simulink library "OSEM_WD"  (Simulink 7.5)
settings: Solver=ode45  StartTime=0.0  StopTime=10.0  RelTol=1e-3
libraries: cdsFunctionCall x3, cdsEpicsOut x2, cdsTrueRMS x1
settings Model: Creator=controls  LastModifiedBy=controls

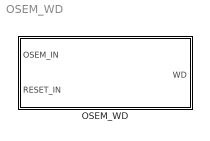
== system OSEM_WD ==
  OSEM_WD : Subsystem

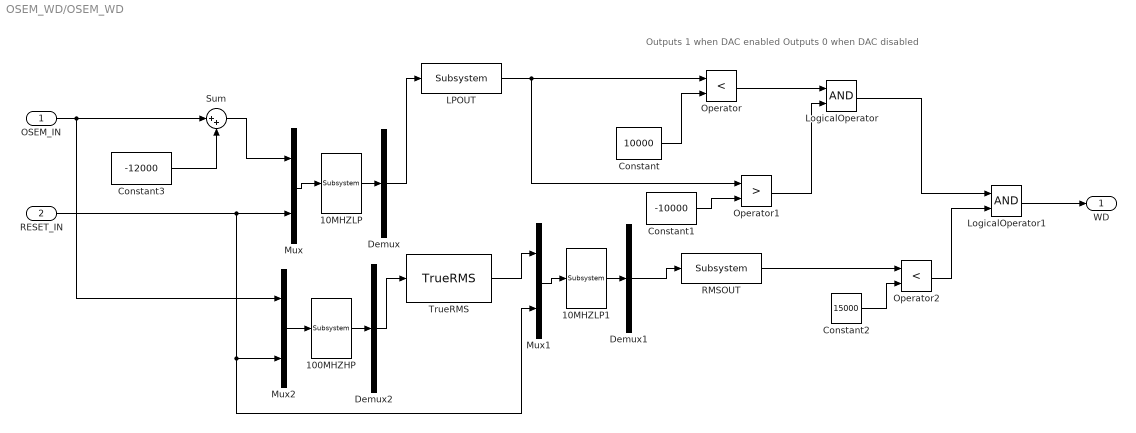
== system OSEM_WD/OSEM_WD ==
  note: Outputs 1 when DAC enabled
      | Outputs 0 when DAC disabled
  OSEM_IN : Inport
  RESET_IN : Inport  Port=2
  100MHZHP : cdsFunctionCall/Subsystem  Tag=cdsFunctionCall  Description=inline FILTER100MHZHP $RCG_DIR/src/drv/susWatchdogFilters.c  SystemSampleTime=-1
      settings: AttributesFormatString=%<Tag>
  10MHZLP : cdsFunctionCall/Subsystem  Tag=cdsFunctionCall  Description=inline FILTER10MHZLP $RCG_DIR/src/drv/susWatchdogFilters.c  SystemSampleTime=-1
      settings: AttributesFormatString=%<Tag>
  10MHZLP1 : cdsFunctionCall/Subsystem  Tag=cdsFunctionCall  Description=inline FILTER10MHZLP $RCG_DIR/src/drv/susWatchdogFilters.c  SystemSampleTime=-1
      settings: AttributesFormatString=%<Tag>
  Constant : Constant  Value=10000
  Constant1 : Constant  Value=-10000
  Constant2 : Constant  Value=15000
  Constant3 : Constant  Value=-12000
  Demux : Demux  Outputs=1
  Demux1 : Demux  Outputs=1
  Demux2 : Demux  Outputs=1
  LPOUT : cdsEpicsOut/Subsystem  Tag=cdsEpicsOutput  Description=|  SystemSampleTime=-1
      | Purpose:                                          
      | Output a FE signal to an EPICS channel.           
      |                                                   
      | Operation:                                        
      | Takes input value and passes it to EPICS record.  
      |                                                   
      | Usage:                                            
      | Name the part with the desired EPICS rrecord name.
      settings: AttributesFormatString=%<Tag>
  LogicalOperator : Logic  AllPortsSameDT=off  OutDataTypeMode=boolean  OutDataTypeStr=boolean
  LogicalOperator1 : Logic  AllPortsSameDT=off  OutDataTypeMode=boolean  OutDataTypeStr=boolean
  Mux : Mux  Inputs=2
  Mux1 : Mux  Inputs=2
  Mux2 : Mux  Inputs=2
  Operator : RelationalOperator  Operator=<  LogicOutDataTypeMode=boolean  OutDataTypeStr=boolean
  Operator1 : RelationalOperator  Operator=>  LogicOutDataTypeMode=boolean  OutDataTypeStr=boolean
  Operator2 : RelationalOperator  Operator=<  LogicOutDataTypeMode=boolean  OutDataTypeStr=boolean
  RMSOUT : cdsEpicsOut/Subsystem  Tag=cdsEpicsOutput  Description=|  SystemSampleTime=-1
      | Purpose:                                          
      | Output a FE signal to an EPICS channel.           
      |                                                   
      | Operation:                                        
      | Takes input value and passes it to EPICS record.  
      |                                                   
      | Usage:                                            
      | Name the part with the desired EPICS rrecord name.
      settings: AttributesFormatString=%<Tag>
  Sum : Sum  Inputs=|++
  TrueRMS : cdsTrueRMS/TrueRMS  Tag=cdsTrueRMS  Description=window_size=655360  SystemSampleTime=-1
      settings: AttributesFormatString=%<Description>\n%<Tag>
  WD : Outport
  wires:
  LogicalOperator1/1 -> WD/1
  Operator2/1 -> LogicalOperator1/2
  LogicalOperator/1 -> LogicalOperator1/1
  Operator1/1 -> LogicalOperator/2
  Operator/1 -> LogicalOperator/1
  Demux/1 -> LPOUT/1
  TrueRMS/1 -> Mux1/1
  10MHZLP/1 -> Demux/1
  Mux/1 -> 10MHZLP/1
  10MHZLP1/1 -> Demux1/1
  Mux1/1 -> 10MHZLP1/1
  Demux1/1 -> RMSOUT/1
  100MHZHP/1 -> Demux2/1
  Mux2/1 -> 100MHZHP/1
  Demux2/1 -> TrueRMS/1
  Constant/1 -> Operator/2
  Constant2/1 -> Operator2/2
  Constant1/1 -> Operator1/2
  RMSOUT/1 -> Operator2/1
  LPOUT/1 -> Operator/1, Operator1/1
  RESET_IN/1 -> Mux/2, Mux2/2, Mux1/2
  Sum/1 -> Mux/1
  Constant3/1 -> Sum/2
  OSEM_IN/1 -> Sum/1, Mux2/1
